simulink model "Powertrain_CheckMate_ver"  (Simulink 7.6)
settings: Solver=ode45  StartTime=0.0  StopTime=60  FixedStep=1e-2
libraries: cmlib x17
settings Model: Creator=yannapur  LastModifiedBy=Georgios
settings DataIOCC: LimitDataPoints=off  SaveOutput=off  SaveState=on  SignalLogging=off
settings DebuggingCC: SolverPrmCheckMsg=none  StrictBusMsg=Warning
settings SFSimCC: SimParseCustomCode=off

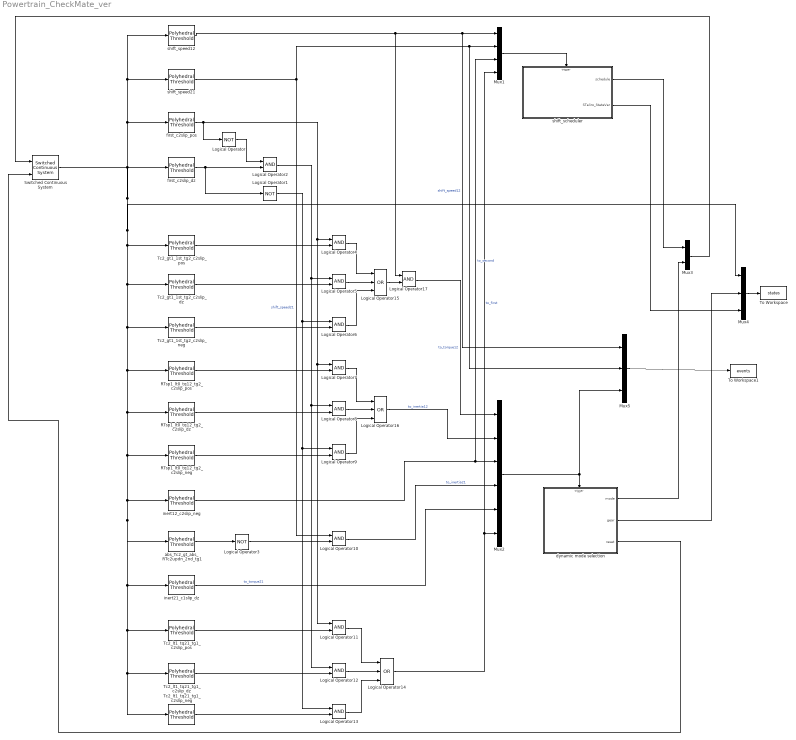
== system Powertrain_CheckMate_ver ==
  Logical Operator : Logic  Operator=NOT
  Logical Operator1 : Logic  Operator=NOT
  Logical Operator{2,4..13,17} (12 alike) : Logic
  Logical Operator14 : Logic  Operator=OR  Inputs=3
  Logical Operator15 : Logic  Operator=OR  Inputs=3
  Logical Operator16 : Logic  Operator=OR  Inputs=3
  Logical Operator3 : Logic  Operator=NOT
  Mux1 : Mux
  Mux2 : Mux  Inputs=6
  Mux3 : Mux  Inputs=2
  Mux4 : Mux  Inputs=3
  Mux5 : Mux  Inputs=3
  RTsp1_lt0_tq12_tg2_c2slip_dz : cmlib/Polyhedral Threshold  SystemSampleTime=-1  polyhedron=RTsp1_lt0_tq12_tg2_c2slip_dz
  RTsp1_lt0_tq12_tg2_c2slip_neg : cmlib/Polyhedral Threshold  SystemSampleTime=-1  polyhedron=RTsp1_lt0_tq12_tg2_c2slip_neg
  RTsp1_lt0_tq12_tg2_c2slip_pos : cmlib/Polyhedral Threshold  SystemSampleTime=-1  polyhedron=RTsp1_lt0_tq12_tg2_c2slip_pos
  Switched Continuous System : cmlib/Switched Continuous System  nx=6  use_sd=off  nup=[]  nz=[]  use_reset=on  nu=2  x0=[0;0;0;0;0;0]  swfunc=hsprb_dynamics  ICS=hsprb_ICS  AR=hsprb_AR  use_param=off  p0=[]  PaCs=[]
  Tc2_gt1_1st_tg2_c2slip_dz : cmlib/Polyhedral Threshold  SystemSampleTime=-1  polyhedron=Tc2_gt1_1st_tg2_c2slip_dz
  Tc2_gt1_1st_tg2_c2slip_neg : cmlib/Polyhedral Threshold  SystemSampleTime=-1  polyhedron=Tc2_gt1_1st_tg2_c2slip_neg
  Tc2_gt1_1st_tg2_c2slip_pos : cmlib/Polyhedral Threshold  SystemSampleTime=-1  polyhedron=Tc2_gt1_1st_tg2_c2slip_pos
  Tc2_lt1_tq21_tg1_c2slip_dz : cmlib/Polyhedral Threshold  SystemSampleTime=-1  polyhedron=Tc2_lt1_tq21_tg1_c2slip_dz
  Tc2_lt1_tq21_tg1_c2slip_neg : cmlib/Polyhedral Threshold  SystemSampleTime=-1  polyhedron=Tc2_lt1_tq21_tg1_c2slip_neg
  Tc2_lt1_tq21_tg1_c2slip_pos : cmlib/Polyhedral Threshold  SystemSampleTime=-1  polyhedron=Tc2_lt1_tq21_tg1_c2slip_pos
  To Workspace : ToWorkspace  VariableName=states  SampleTime=-1  SaveFormat=Structure
  To Workspace1 : ToWorkspace  VariableName=events  SampleTime=-1  SaveFormat=Structure
  abs_Tc2_gt_abs_RTc2updn_2nd_tg1 : cmlib/Polyhedral Threshold  SystemSampleTime=-1  polyhedron=abs_Tc2_gt_abs_RTc2updn_2nd_tg1
  dynamic mode selection : Stateflow chart  TreatAsAtomicUnit=on
  first_c2slip_dz : cmlib/Polyhedral Threshold  SystemSampleTime=-1  polyhedron=first_c2slip_dz
  first_c2slip_pos : cmlib/Polyhedral Threshold  SystemSampleTime=-1  polyhedron=first_c2slip_pos
  inert12_c2slip_neg : cmlib/Polyhedral Threshold  SystemSampleTime=-1  polyhedron=inert12_c2slip_neg
  inert21_c1slip_dz : cmlib/Polyhedral Threshold  SystemSampleTime=-1  polyhedron=inert21_c1slip_dz
  shift_scheduler : Stateflow chart  TreatAsAtomicUnit=on
  shift_speed12 : cmlib/Polyhedral Threshold  SystemSampleTime=-1  polyhedron=shift_speed12
  shift_speed21 : cmlib/Polyhedral Threshold  SystemSampleTime=-1  polyhedron=shift_speed21
  wires:
  Switched Continuous System/1 -> shift_speed12/1, shift_speed21/1, first_c2slip_pos/1, first_c2slip_dz/1, Tc2_gt1_1st_tg2_c2slip_pos/1, Tc2_gt1_1st_tg2_c2slip_dz/1, Tc2_gt1_1st_tg2_c2slip_neg/1, RTsp1_lt0_tq12_tg2_c2slip_pos/1, RTsp1_lt0_tq12_tg2_c2slip_dz/1, RTsp1_lt0_tq12_tg2_c2slip_neg/1, inert12_c2slip_neg/1, abs_Tc2_gt_abs_RTc2updn_2nd_tg1/1, inert21_c1slip_dz/1, Tc2_lt1_tq21_tg1_c2slip_pos/1, Tc2_lt1_tq21_tg1_c2slip_dz/1, Tc2_lt1_tq21_tg1_c2slip_neg/1, Mux4/1
  Logical Operator/1 -> Logical Operator2/1
  first_c2slip_dz/1 -> Logical Operator2/2, Logical Operator1/1
  Tc2_gt1_1st_tg2_c2slip_pos/1 -> Logical Operator4/2
  Tc2_gt1_1st_tg2_c2slip_dz/1 -> Logical Operator5/2
  Tc2_gt1_1st_tg2_c2slip_neg/1 -> Logical Operator6/2
  RTsp1_lt0_tq12_tg2_c2slip_pos/1 -> Logical Operator7/2
  RTsp1_lt0_tq12_tg2_c2slip_dz/1 -> Logical Operator8/2
  RTsp1_lt0_tq12_tg2_c2slip_neg/1 -> Logical Operator9/2
  abs_Tc2_gt_abs_RTc2updn_2nd_tg1/1 -> Logical Operator3/1
  Logical Operator3/1 -> Logical Operator10/2
  Tc2_lt1_tq21_tg1_c2slip_pos/1 -> Logical Operator11/2
  Tc2_lt1_tq21_tg1_c2slip_dz/1 -> Logical Operator12/2
  Tc2_lt1_tq21_tg1_c2slip_neg/1 -> Logical Operator13/2
  first_c2slip_pos/1 -> Logical Operator4/1, Logical Operator11/1, Logical Operator7/1, Logical Operator/1
  Logical Operator2/1 -> Logical Operator5/1, Logical Operator12/1, Logical Operator8/1
  Logical Operator1/1 -> Logical Operator6/1, Logical Operator13/1, Logical Operator9/1
  shift_speed21/1 -> Logical Operator10/1, Mux1/2, Mux5/2  "shift_speed21"
  Logical Operator11/1 -> Logical Operator14/1
  Logical Operator12/1 -> Logical Operator14/2
  Logical Operator13/1 -> Logical Operator14/3
  Logical Operator7/1 -> Logical Operator16/1
  Logical Operator8/1 -> Logical Operator16/2
  Logical Operator9/1 -> Logical Operator16/3
  Logical Operator4/1 -> Logical Operator15/1
  Logical Operator5/1 -> Logical Operator15/2
  Logical Operator6/1 -> Logical Operator15/3
  Logical Operator15/1 -> Logical Operator17/2
  shift_speed12/1 -> Logical Operator17/1, Mux1/1, Mux5/1  "shift_speed12"
  Logical Operator14/1 -> Mux1/4, Mux2/6  "to_first"
  Logical Operator17/1 -> Mux2/1  "to_torque12"
  Logical Operator16/1 -> Mux2/2  "to_inertia12"
  inert12_c2slip_neg/1 -> Mux1/3, Mux2/3  "to_second"
  Logical Operator10/1 -> Mux2/4  "to_inertia21"
  inert21_c1slip_dz/1 -> Mux2/5  "to_torque21"
  Mux3/1 -> Switched Continuous System/1
  Mux2/1 -> dynamic mode selection/Trigger, Mux5/3
  Mux4/1 -> To Workspace/1
  Mux1/1 -> shift_scheduler/Trigger
  shift_scheduler/1(schedule) -> Mux3/1
  dynamic mode selection/1(mode) -> Mux3/2
  dynamic mode selection/3(reset) -> Switched Continuous System/2
  Mux5/1 -> To Workspace1/1
  dynamic mode selection/2(gear) -> Mux4/2
  shift_scheduler/2(STaliro_StateVar) -> Mux4/3

== stateflow chart shift_scheduler ==
  settings: executeAtInitialization=1
  state first_gear
    entry: schedule =1;
    STaliro_StateVar = 1;
  state transition21_shifting
    entry:schedule = 4;
    STaliro_StateVar = 4;
  state second_gear
    entry: schedule =3;
    STaliro_StateVar = 3;
  state transition12_shifting
    entry : schedule = 2;
    STaliro_StateVar = 2;
  transition12_shifting -> second_gear [order 1] : to_second
  second_gear -> transition21_shifting : shift_speed21
  transition21_shifting -> second_gear [order 2] : shift_speed12
  transition21_shifting -> first_gear [order 1] : to_first
  first_gear -> transition12_shifting : shift_speed12
  transition12_shifting -> first_gear [order 2] : shift_speed21
  (default) -> first_gear
  data: schedule output double =1; STaliro_StateVar output double
  events: shift_speed12 input RISING_EDGE_EVENT; shift_speed21 input RISING_EDGE_EVENT; to_second input RISING_EDGE_EVENT; to_first input RISING_EDGE_EVENT

== stateflow chart dynamic mode selection ==
  state first
    entry: mode = 1;
    gear = 1;
  state torque12
    entry:mode = 2;
    gear=1.5;
  state torque21
    entry:mode = 6;
    gear=1.5;
  state inertia12
    entry: mode=3;
    gear=1.5;
  state inertia21
    entry:mode = 5;
    gear=1.5;
  state second
    entry: mode = 4;
    gear=2;
  (default) -> first
  torque21 -> first : to_first
  first -> torque12 : to_torque12
  torque12 -> inertia12 : to_inertia12
  second -> inertia21 : to_inertia21
  inertia21 -> torque21 : to_torque21/reset;
  inertia12 -> second : to_second/reset;
  data: mode output double =1; gear output double =1
  events: to_torque12 input RISING_EDGE_EVENT; to_inertia12 input RISING_EDGE_EVENT; to_second input RISING_EDGE_EVENT; to_inertia21 input RISING_EDGE_EVENT; to_torque21 input RISING_EDGE_EVENT; to_first input RISING_EDGE_EVENT; reset output EITHER_EDGE_EVENT
